simulink model "Offline_DataImport"  (R2019a)
settings: Solver=FixedStepDiscrete  StartTime=0.0  StopTime=param_sim_time  FixedStep=1/fs  MaxStep=1/fs  RelTol=1e-3
undefined symbols (not defined in the file): fs, param_tot_samples
settings Model: PacingRate=100  Creator=rcord  LastModifiedBy=rcord
settings SolverCC: ZeroCrossControl=DisableAll
settings DataIOCC: ExternalInput=[t, signals.ecg.input, signals.scg.input_x, signals.scg.input_y, signals.scg.input_z]  LoadExternalInput=on  SignalLogging=off  DSMLogging=off  SaveTime=off  ReturnWorkspaceOutputs=off  TimeSaveName=t_preprocessing  OutputSaveName=out_preprocessing  LoggingIntervals=[-inf,inf]

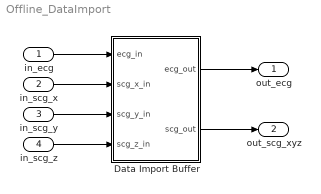
== system Offline_DataImport ==
  in_ecg : Inport  SampleTime=1/fs
  in_scg_x : Inport  Port=2  SampleTime=1/fs
  in_scg_y : Inport  Port=3  SampleTime=1/fs
  in_scg_z : Inport  Port=4  SampleTime=1/fs
  Data Import Buffer : Subsystem
  out_ecg : Outport
  out_scg_xyz : Outport  Port=2
  wires:
  in_ecg/1 -> Data Import Buffer/1(ecg_in)
  in_scg_x/1 -> Data Import Buffer/2(scg_x_in)
  in_scg_y/1 -> Data Import Buffer/3(scg_y_in)
  in_scg_z/1 -> Data Import Buffer/4(scg_z_in)
  Data Import Buffer/1(ecg_out) -> out_ecg/1
  Data Import Buffer/2(scg_out) -> out_scg_xyz/1

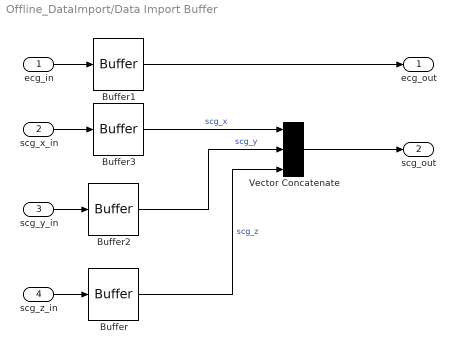
== system Offline_DataImport/Data Import Buffer ==
  ecg_in : Inport
  scg_x_in : Inport  Port=2
  scg_y_in : Inport  Port=3
  scg_z_in : Inport  Port=4
  Buffer{,1..3} (4 alike) : Buffer  N=param_tot_samples  OutputFrames=off
  Vector Concatenate : Concatenate  NumInputs=3  Mode=Multidimensional array  ConcatenateDimension=2
  ecg_out : Outport
  scg_out : Outport  Port=2
  wires:
  ecg_in/1 -> Buffer1/1
  Buffer/1 -> Vector Concatenate/3  "scg_z"
  Buffer3/1 -> Vector Concatenate/1  "scg_x"
  scg_x_in/1 -> Buffer3/1
  Vector Concatenate/1 -> scg_out/1
  Buffer1/1 -> ecg_out/1
  Buffer2/1 -> Vector Concatenate/2  "scg_y"
  scg_z_in/1 -> Buffer/1
  scg_y_in/1 -> Buffer2/1
